simulink model "pendule_simple"  (R2016a)
settings: Solver=VariableStepAuto  StartTime=0.0  StopTime=100.0  RelTol=1e-3
undefined symbols (not defined in the file): K
libraries: simulink x1
settings Model: Creator=tmeunier  LastModifiedBy=tmeunier

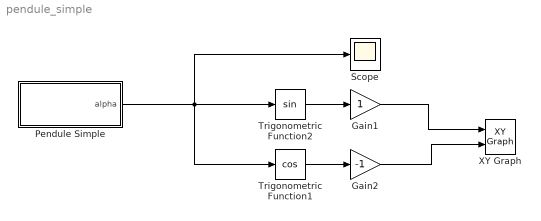
== system pendule_simple ==
  Gain1 : Gain
  Gain2 : Gain  Gain=-1
  Pendule Simple : Subsystem
  Scope : Scope
  Trigonometric Function1 : Trigonometry  Operator=cos
  Trigonometric Function2 : Trigonometry
  XY Graph : simulink/Sinks/XY Graph  xmin=-1  xmax=1  ymin=-1  ymax=1  st=-1
  wires:
  Gain1/1 -> XY Graph/1
  Trigonometric Function2/1 -> Gain1/1
  Trigonometric Function1/1 -> Gain2/1
  Gain2/1 -> XY Graph/2
  Pendule Simple/1(alpha) -> Scope/1, Trigonometric Function1/1, Trigonometric Function2/1

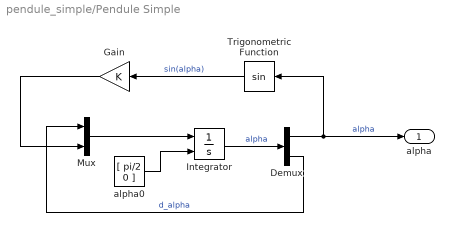
== system pendule_simple/Pendule Simple ==
  Demux : Demux  Outputs=2
  Gain : Gain  Gain=K
  Integrator : Integrator  InitialConditionSource=external
  Mux : Mux  Inputs=2
  Trigonometric Function : Trigonometry
  alpha0 : Constant  Value=[ pi/2 0 ]
  alpha : Outport
  wires:
  Trigonometric Function/1 -> Gain/1  "sin(alpha)"
  alpha0/1 -> Integrator/2
  Integrator/1 -> Demux/1  "alpha"
  Demux/1 -> Trigonometric Function/1, alpha/1  "alpha"
  Demux/2 -> Mux/1  "d_alpha"
  Gain/1 -> Mux/2
  Mux/1 -> Integrator/1
